simulink model "ProgrammablePulseGenerator"  (Simulink 7.1)
settings: Solver=ode45  StartTime=0.0  StopTime=10.0  RelTol=1e-3
libraries: simulink x1
settings Model: Creator=lid  LastModifiedBy=lid

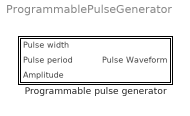
== system ProgrammablePulseGenerator ==
  Programmable pulse generator : Subsystem

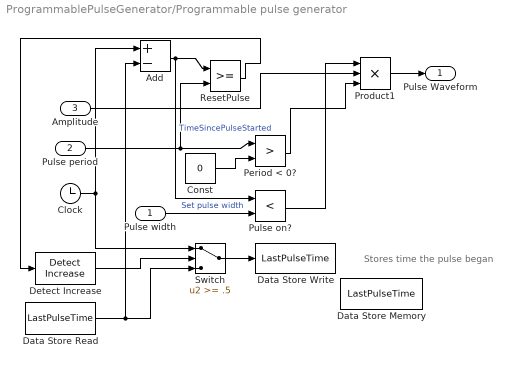
== system ProgrammablePulseGenerator/Programmable pulse generator ==
  note: Stores time the pulse began
  Pulse width : Inport  OutDataType=sfix(16)  OutScaling=2^0
  Pulse period : Inport  Port=2  OutDataType=sfix(16)  OutScaling=2^0
  Amplitude : Inport  Port=3  OutDataType=sfix(16)  OutScaling=2^0
  Add : Sum  Inputs=+-  OutDataType=sfix(16)  OutScaling=2^-10
  Clock : Clock
      settings: Decimation=10
  Const : Constant  Value=0  OutDataType=sfix(16)  OutScaling=2^0
  Data Store Memory : DataStoreMemory  DataStoreName=LastPulseTime  OutDataType=sfix(16)  OutScaling=2^0
  Data Store Read : DataStoreRead  DataStoreName=LastPulseTime  SampleTime=0
  Data Store Write : DataStoreWrite  DataStoreName=LastPulseTime  SampleTime=-1
  Detect Increase : simulink/Logic and Bit Operations/Detect Increase  SystemSampleTime=-1  vinit=0.0
  Period < 0? : RelationalOperator  Operator=>  LogicOutDataTypeMode=boolean  OutDataTypeStr=boolean
  Product1 : Product  Inputs=3  OutDataType=sfix(16)  OutScaling=2^0  RndMeth=Zero
  Pulse on? : RelationalOperator  Operator=<  LogicOutDataTypeMode=boolean  OutDataTypeStr=boolean
  ResetPulse : RelationalOperator  LogicOutDataTypeMode=boolean  OutDataTypeStr=boolean
  Switch : Switch  Threshold=.5  OutDataType=sfix(16)  OutScaling=2^0
  Pulse Waveform : Outport  OutDataType=sfix(16)  OutScaling=2^0
  wires:
  Pulse period/1 -> Period < 0?/1, ResetPulse/2
  Clock/1 -> Add/1, Switch/1
  ResetPulse/1 -> Detect Increase/1
  Product1/1 -> Pulse Waveform/1
  Amplitude/1 -> Product1/2
  Period < 0?/1 -> Product1/3
  Const/1 -> Period < 0?/2
  Switch/1 -> Data Store Write/1
  Data Store Read/1 -> Add/2, Switch/3
  Detect Increase/1 -> Switch/2
  Add/1 -> ResetPulse/1, Pulse on?/1  "TimeSincePulseStarted"
  Pulse on?/1 -> Product1/1
  Pulse width/1 -> Pulse on?/2  "Set pulse width"
